simulink model "park"  (R2022b)
settings: Solver=VariableStepAuto  StartTime=0.0  StopTime=10.0  RelTol=1e-3
settings Model: Creator=15403  LastModifiedBy=15403

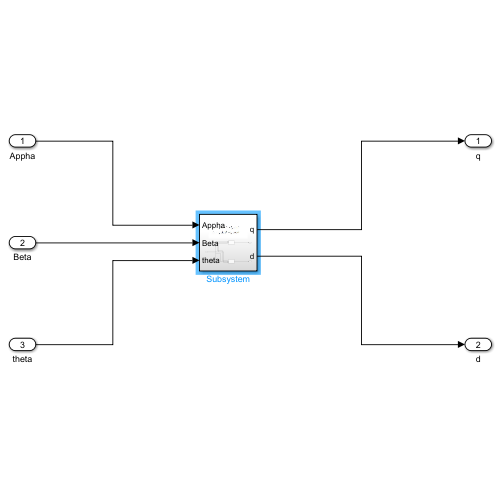
[thumbnail: Simulink's stored preview of the top-level diagram]
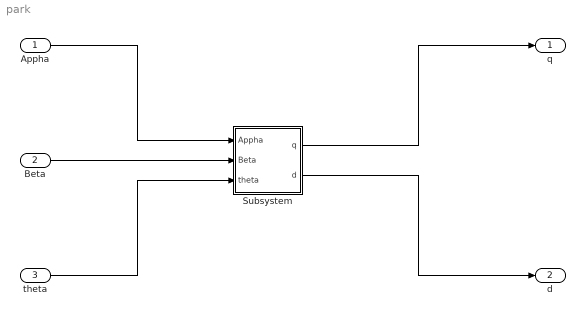
== system park ==
  Appha : Inport
  Beta : Inport  Port=2
  theta : Inport  Port=3
  Subsystem : Subsystem
  q : Outport
  d : Outport  Port=2
  wires:
  Appha/1 -> Subsystem/1(Appha)
  Beta/1 -> Subsystem/2(Beta)
  theta/1 -> Subsystem/3(theta)
  Subsystem/1(q) -> q/1
  Subsystem/2(d) -> d/1

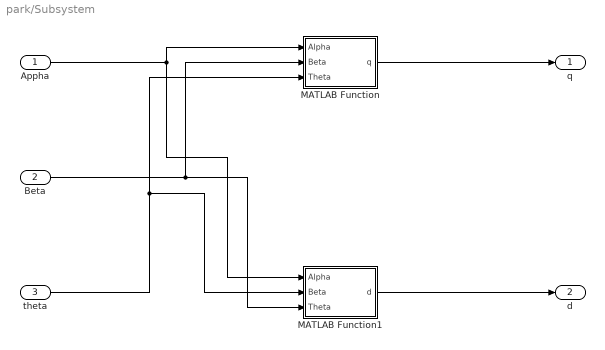
== system park/Subsystem ==
  Appha : Inport
  Beta : Inport  Port=2
  theta : Inport  Port=3
  MATLAB Function : MATLAB Function  TreatAsAtomicUnit=on
  MATLAB Function1 : MATLAB Function  TreatAsAtomicUnit=on
  q : Outport
  d : Outport  Port=2
  wires:
  theta/1 -> MATLAB Function1/2(Beta), MATLAB Function/3(Theta)
  MATLAB Function1/1(d) -> d/1
  Beta/1 -> MATLAB Function1/3(Theta), MATLAB Function/2(Beta)
  Appha/1 -> MATLAB Function1/1(Alpha), MATLAB Function/1(Alpha)
  MATLAB Function/1(q) -> q/1

== matlab function park/Subsystem/MATLAB Function ==
  data: Alpha input; q output; Beta input; Theta input
function q = fcn(Alpha, Beta, Theta)

q = Alpha * cosd(Theta) - Beta * sind(Theta);

== matlab function park/Subsystem/MATLAB Function1 ==
  data: Alpha input; d output; Beta input; Theta input
function d = fcn(Alpha, Beta, Theta)

d = Alpha * sind(Theta) + Beta * cosd(Theta);
